simulink subsystem "Encoder"  (R2022b)
settings: Solver=VariableStepAuto  StartTime=0.0  StopTime=10.0  RelTol=1e-3
libraries: simulink x1
settings Model: Creator=Usuario  LastModifiedBy=Usuario
settings OptimizationCC: ReuseModelBlockBuffer=on
settings RTWCC: GPUComputeCapability=5.0

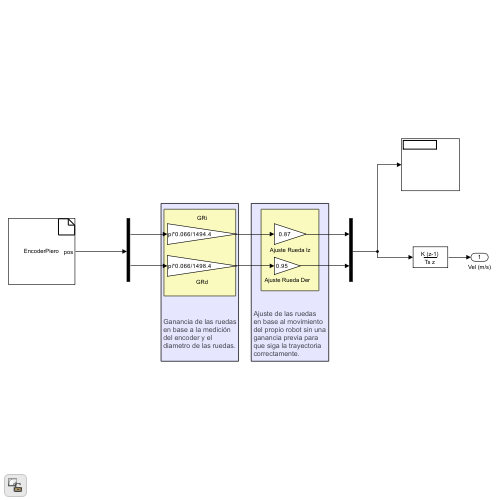
[thumbnail: Simulink's stored preview of the top-level diagram]
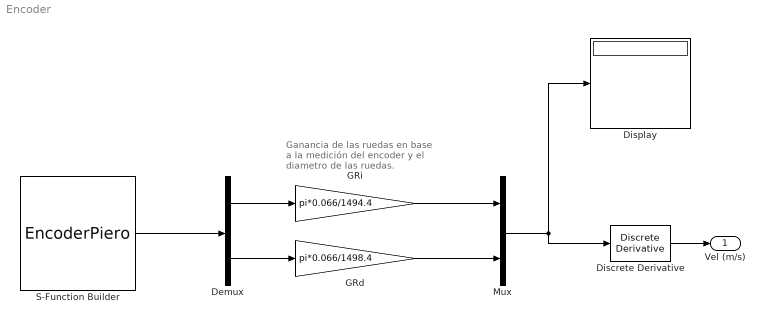
== system Encoder ==
  note: Ganancia de las ruedas
      | en base a la medición
      | del encoder y el
      | diametro de las ruedas.
  Demux : Demux  Outputs=2
  Discrete Derivative : simulink/Discrete/Discrete Derivative  gainval=1.0  ICPrevScaledInput=0.0  OutMin=[]  OutMax=[]  OutDataTypeStr=double  OutputDataTypeScalingMode=double  OutDataType=fixdt(1, 16)  OutScaling=2^-10  DoSatur=off
  Display : Display
  GRd : Gain  Gain=pi*0.066/1498.4
  GRi : Gain  Gain=pi*0.066/1494.4
  Mux : Mux  Inputs=2
  S-Function Builder : S-Function  FunctionName=EncoderPiero  SFunctionModules=EncoderPiero_wrapper.c  SFunctionDeploymentMode=off  EnableBusSupport=off  mask(S-Function Builder){}
      mask help: Simulink:masks:SFunctionBuilder_MD
      mask init:
      | val = [[.9  0.75 0.75 1 1 .9 .9 1]',[1 1 0.75 0.75 .9 .9 1 .9]'];try , sys = get_param(gcb,'SfunBuilderFcnName');if isempty(sys), sys = get_param(gcb,'FunctionName'); end,catch, sys = get_param(gcb,'FunctionName'); end
      settings: CopyFcn=set_param(gcbh,'LinkStatus','none')  OpenFcn=sfunctionwizard(gcbh)
      mask Display:
      | plot(val(:,1),val(:,2))
      | disp(sys)
      | port_label('output',1,sprintf('%s', 'pos'),'interpreter','tex')
  Vel (m/s) : Outport
  wires:
  Discrete Derivative/1 -> Vel (m/s)/1
  Mux/1 -> Discrete Derivative/1, Display/1
  Demux/2 -> GRd/1
  Demux/1 -> GRi/1
  S-Function Builder/1 -> Demux/1
  GRi/1 -> Mux/1
  GRd/1 -> Mux/2
